simulink model "myTV_MPCC_fix"  (R2023b)
settings: Solver=VariableStepAuto  StartTime=0.0  StopTime=10.0  FixedStep=1e-6  RelTol=1e-3
libraries: spsDCVoltageSourceLib x1, slpidlib x1, spsPermanentMagnetSynchronousMachineLib x1, spsUniversalBridgeLib x1, spspowerguiLib x1
settings Model: Creator=XieXW  LastModifiedBy=XieXW
settings ModelReferenceCC: EnableRefExpFcnMdlSchedulingChecks=on

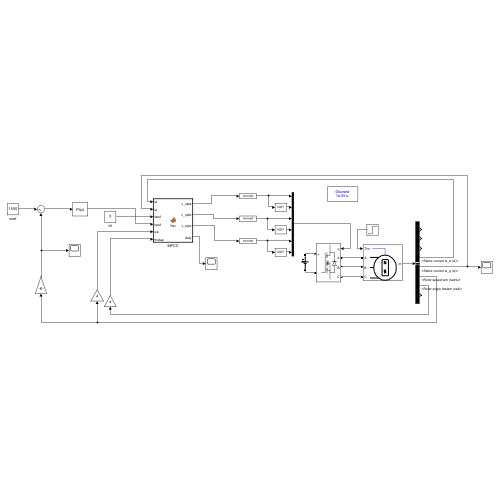
[thumbnail: Simulink's stored preview of the top-level diagram]
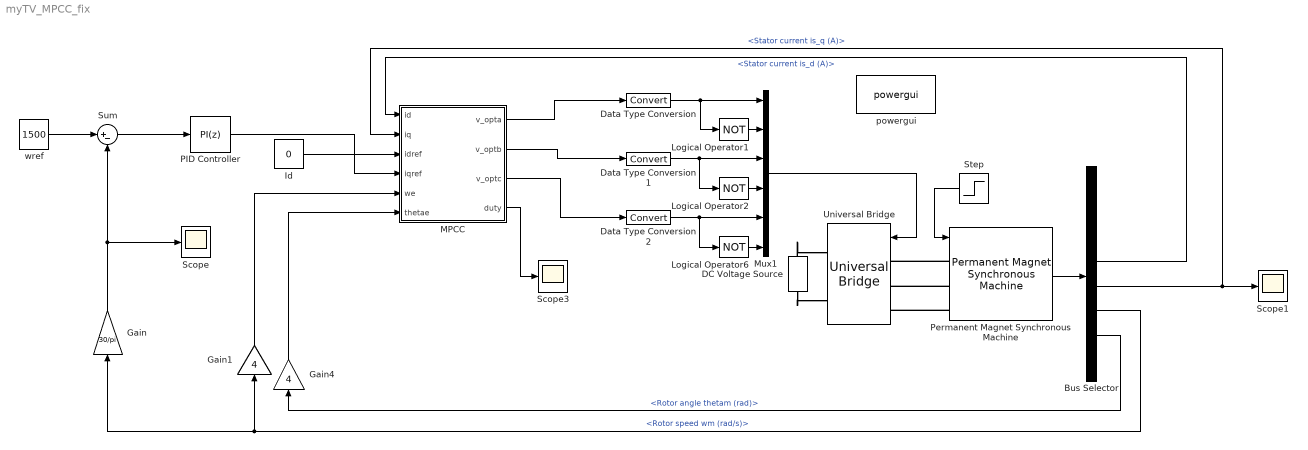
== system myTV_MPCC_fix ==
  Bus Selector : BusSelector  OutputSignals=Stator current is_a (A),Stator current is_b (A),Stator current is_c (A),Stator current is_d (A),Stator current is_q (A),Rotor speed wm (rad/s),Rotor angle thetam (rad),Electromagnetic torque Te (N*m)
  DC Voltage Source : spsDCVoltageSourceLib/DC Voltage Source  Amplitude=24  Measurements=None
  Data Type Conversion : DataTypeConversion  SaturateOnIntegerOverflow=off  RndMeth=Floor
  Data Type Conversion1 : DataTypeConversion  SaturateOnIntegerOverflow=off  RndMeth=Floor
  Data Type Conversion2 : DataTypeConversion  SaturateOnIntegerOverflow=off  RndMeth=Floor
  Gain : Gain  Gain=30/pi
  Gain1 : Gain  Gain=4
  Gain4 : Gain  Gain=4
  Id : Constant  Value=0
  Logical Operator1 : Logic  Operator=NOT  AllPortsSameDT=off  OutDataTypeStr=boolean
  Logical Operator2 : Logic  Operator=NOT  AllPortsSameDT=off  OutDataTypeStr=boolean
  Logical Operator6 : Logic  Operator=NOT  AllPortsSameDT=off  OutDataTypeStr=boolean
  MPCC : MATLAB Function  TreatAsAtomicUnit=on
  Mux1 : Mux  Inputs=6
  PID Controller : slpidlib/PID Controller  Controller=PI  Form=Parallel  TimeDomain=Discrete-time  UseExternalTs=off  SampleTime=-1  IntegratorMethod=Forward Euler  FilterMethod=Forward Euler  ControllerParametersSource=internal  P=0.6  I=0.7  UseKiTs=off  D=0  N=100  UseFilter=on  TunerSelectOption=Transfer Function Based (PID Tuner App)  InitialConditionSource=internal  InitialConditionForIntegrator=0  InitialConditionForFilter=0  DifferentiatorICPrevScaledInput=0  ExternalReset=none  TrackingMode=off  Kt=1  LimitOutput=off  SatLimitsSource=internal  UpperSaturationLimit=inf  LowerSaturationLimit=-inf  LinearizeAsGain=on  AntiWindupMode=none  Kb=1  LimitIntegrator=off  UpperIntegratorSaturationLimit=inf  LowerIntegratorSaturationLimit=-inf  POutMin=[]  POutMax=[]  IOutMin=[]  IOutMax=[]  DOutMin=[]  DOutMax=[]  NOutMin=[]  NOutMax=[]  SumOutMin=[]  SumOutMax=[]  SaturationOutMin=[]  SaturationOutMax=[]  PParamMin=[]  PParamMax=[]  IParamMin=[]  IParamMax=[]  DParamMin=[]  DParamMax=[]  NParamMin=[]  NParamMax=[]  KbParamMin=[]  KbParamMax=[]  KtParamMin=[]  KtParamMax=[]  KbOutMin=[]  KbOutMax=[]  KtOutMin=[]  KtOutMax=[]  IntegratorOutMin=[]  IntegratorOutMax=[]  FilterOutMin=[]  FilterOutMax=[]  SumI1OutMin=[]  SumI1OutMax=[]  SumI2OutMin=[]  SumI2OutMax=[]  SumI3OutMin=[]  SumI3OutMax=[]  SumI4OutMin=[]  SumI4OutMax=[]  SumDOutMin=[]  SumDOutMax=[]  DifferentiatorOutMin=[]  DifferentiatorOutMax=[]  FilterDiffOutCoefMin=[]  FilterDiffOutCoefMax=[]  ReciprocalOutMin=[]  ReciprocalOutMax=[]  SumDenOutMin=[]  SumDenOutMax=[]  SumNumOutMin=[]  SumNumOutMax=[]  DivideOutMin=[]  DivideOutMax=[]  UdiffTsProdOutMin=[]  UdiffTsProdOutMax=[]  NTsProdOutMin=[]  NTsProdOutMax=[]  UintegralTsProdOutMin=[]  UintegralTsProdOutMax=[]  UngainTsProdOutMin=[]  UngainTsProdOutMax=[]  ClampingZeroOutDataTypeStr=Inherit: Inherit via back propagation  ClampingZeroOutMin=[]  ClampingZeroOutMax=[]  FilterDenConstantOutDataTypeStr=Inherit: Inherit via back propagation  FilterDenConstantOutMin=[]  FilterDenConstantOutMax=[]  PCopyOutDataTypeStr=Inherit: Inherit via back propagation  PCopyOutMin=[]  PCopyOutMax=[]  NCopyOutDataTypeStr=Inherit: Inherit via back propagation  NCopyOutMin=[]  NCopyOutMax=[]  IntegratorContinuousStateAttributes=''  IntegratorStateMustResolveToSignalObject=off  IntegratorRTWStateStorageClass=Auto  FilterContinuousStateAttributes=''  FilterStateMustResolveToSignalObject=off  FilterRTWStateStorageClass=Auto  ParallelPVariant=InternalParameters  IdealPVariant=Disabled  IVariant=InternalParameters  DVariant=Disabled  IntegratorVariant=Discrete  SatVariant=Disabled  AWVariant=Passthrough  PCopyVariant=Disabled  TRVariant=Disabled  FdbkBlocksVariant=Forward  IdealPFdbkVariant=Disabled  SatFdbkVariant=Disabled  DerivativeFilterVariant=Disabled  NVariant=Disabled  NCopyVariant=Disabled_SignalSpec  FilterICVariant=Disabled  IntegratorICVariant=InternalICs  ExternalResetVariant=Disabled  TRSumVariant=Passthrough  SumFdbkVariant=Disabled  SumVariant=Sum_PI  TsampFilterVariant=InternalTs  TsampNgainVariant=Passthrough  TsampIntegralVariant=Disabled_SignalSpec  ExternalSaturationOutDataTypeStr=Inherit: Same as second input
  Permanent Magnet Synchronous Machine : spsPermanentMagnetSynchronousMachineLib/Permanent Magnet Synchronous Machine  NbPhases=3  FluxDistribution=Sinusoidal  RotorType=Round  MechanicalLoad=Torque Tm  PresetModel=No  ShowDetailedParameters=on  MeasurementBus=off  Resistance=0.03  Inductance=8.5e-3  dqInductances=[8.5e-3,8.5e-3]  La=0.00015  MachineConstant=Flux linkage established by magnets (V.s)  Flux=0.008  VoltageCst=5.8042  TorqueCst=0.048  Flat=120  Mechanical=[0.0027 0.0004924 4 0]  PolePairs=4  InitialConditions=[0,0, 0,0]  InitialConditions5ph=[0 0 0 0 0 0]  RefAngle=Aligned with phase A axis (original Park)  IterativeDiscreteModel=Trapezoidal non iterative  TsBlock=-1  TsPowergui=0
  Scope : Scope
  Scope1 : Scope
  Scope3 : Scope
  Step : Step  Time=5  After=2  SampleTime=0
  Sum : Sum  Inputs=|+-
  Universal Bridge : spsUniversalBridgeLib/Universal Bridge  Arms=3  SnubberResistance=1e5  SnubberCapacitance=inf  Device=MOSFET / Diodes  Ron=1e-3  Lon=0  ForwardVoltages="[  0  0  ]"  ForwardVoltage=0  GTOparameters=[ 10e-6 , 20e-6 ]  IGBTparameters=[ 1e-6 , 2e-6 ]  Measurements=None  Measurements_2=None  converterType=Rectifier
  powergui : spspowerguiLib/powergui  Priority=1  SimulationMode=Discrete  SampleTime=1e-05  frequency=60  Iterations=50  frequencyindice=0  Pbase=100e6  ErrMax=1e-4  UnitsV=kV  UnitsW=MW  buscounter=0  FunctionMessages=off  echomessages=off  EnableUseOfTLC=off  CurrentSourceSwitches=off  DisableSnubberDevices=off  DisableRonSwitches=off  DisableVfSwitches=off  DisplayEquations=off  AutomaticDiscreteSolvers=off  SolverType=Tustin/Backward Euler (TBE)  Interpol=off  ExternalGateDelay=off  methode=off  Ts=100  x0status=blocks  SPID=on  SwTol=0  HookPort=off  NonlinearTolerance=1e-4  nMaxIteration=100  ContinueOnMaxIteration=off  RestoreLinks=warning  ResistiveCurrentMeasurement=off  Frange=[0:2:500]  Ylog=off  Xlog=on  ShowGrid=off  save=off  variable=ZData  structure=0  ZoomFFT=off  StartTime=0.0  cycles=1  DisplayStyle=1  fundamental=60  FreqAxis=off  MaxFrequency=1000  frequencyindicesteady=1  RmsSteady=1  display=off
  wref : Constant  Value=1500
  wires:
  wref/1 -> Sum/1
  Sum/1 -> PID Controller/1
  PID Controller/1 -> MPCC/4(iqref)
  Permanent Magnet Synchronous Machine/1 -> Bus Selector/1
  Bus Selector/4 -> MPCC/1(id)  "<Stator current is_d (A)>"
  Bus Selector/5 -> Scope1/1, MPCC/2(iq)  "<Stator current is_q (A)>"
  Bus Selector/7 -> Gain4/1  "<Rotor angle thetam (rad)>"
  Bus Selector/6 -> Gain/1, Gain1/1  "<Rotor speed wm (rad/s)>"
  Id/1 -> MPCC/3(idref)
  Gain/1 -> Sum/2, Scope/1
  Gain4/1 -> MPCC/6(thetae)
  Gain1/1 -> MPCC/5(we)
  Step/1 -> Permanent Magnet Synchronous Machine/1
  MPCC/2(v_optb) -> Data Type Conversion1/1
  Logical Operator6/1 -> Mux1/6
  Data Type Conversion/1 -> Mux1/1, Logical Operator1/1
  Logical Operator1/1 -> Mux1/2
  Mux1/1 -> Universal Bridge/1
  MPCC/1(v_opta) -> Data Type Conversion/1
  Logical Operator2/1 -> Mux1/4
  Data Type Conversion1/1 -> Mux1/3, Logical Operator2/1
  MPCC/4(duty) -> Scope3/1
  Data Type Conversion2/1 -> Logical Operator6/1, Mux1/5
  MPCC/3(v_optc) -> Data Type Conversion2/1
  connections:
  Permanent Magnet Synchronous Machine/LConn1 -- Universal Bridge/LConn1
  Permanent Magnet Synchronous Machine/LConn2 -- Universal Bridge/LConn2
  Permanent Magnet Synchronous Machine/LConn3 -- Universal Bridge/LConn3
  DC Voltage Source/RConn1 -- Universal Bridge/RConn1
  DC Voltage Source/LConn1 -- Universal Bridge/RConn2

== matlab function myTV_MPCC_fix/MPCC ==
  settings: sampleTime=20e-6
  data: id input; v_opta output; v_optb output; v_optc output; duty output; iq input; idref input; iqref input; we input; thetae input
function [v_opta,v_optb,v_optc,duty] = fcn(id,iq,idref,iqref,we,thetae)

Rs=0.03;
Ls=0.00015;
psif=0.008;
vdc=24;
Ts=1e-4;
set=[0 0 0;0 1 0;0 0 1;0 1 1;1 0 0;1 0 1;1 1 0];%电压矢量开关集合
cost = 1000000;
state1 = 1;
state2 = 1;
%%开始计算第一个最优电压矢量
for i=1:7
    udi=2/3*vdc*( set(i,1)*cos(thetae)+set(i,2)*cos(thetae-2*pi/3)+set(i,3)*cos(thetae+2*pi/3));
    uqi=2/3*vdc*(-set(i,1)*sin(thetae)-set(i,2)*sin(thetae-2*pi/3)-set(i,3)*sin(thetae+2*pi/3));
    id1 = id+Ts/Ls*(udi-Rs*id+we*Ls*iq);
    iq1 = iq+Ts/Ls*(uqi-Rs*iq-we*(Ls*id+psif));

    J = (idref-id1)^2+(iqref-iq1)^2;
    if J<cost
        state1=i;
        cost = J;
    end

end
%%第一个最优电压矢量
v_opt1_a = set(state1,1);
v_opt1_b = set(state1,2);
v_opt1_c = set(state1,3);
v_opt1 = [v_opt1_a,v_opt1_b,v_opt1_c];

%%开始计算第二个最优电压矢量
%计算最优电压矢量
uq_opt1 = 2/3*vdc*( set(state1,1)*cos(thetae)+set(state1,2)*cos(thetae-2*pi/3)+set(state1,3)*cos(thetae+2*pi/3));
ud_opt1 = 2/3*vdc*(-set(state1,1)*sin(thetae)-set(state1,2)*sin(thetae-2*pi/3)-set(state1,3)*sin(thetae+2*pi/3));

slope = [0 0 0 0 0 0 0];                %七个电压矢量作用下的q轴电流斜率
slope_0 = -Rs/Ls*iq-we*id-we*psif/Ls;    %零电压矢量作用下的q轴电流斜率
slope_opt = slope_0 + uq_opt1/Ls;       %最优矢量作用下的q轴电流斜率

%重新初始化代价值
cost = 1000000;

for j=1:7
    %%步骤1
    %计算第j个电压矢量的dq轴分量,对应论文中的uqj、udj
    udj=2/3*vdc*( set(j,1)*cos(thetae)+set(j,2)*cos(thetae-2*pi/3)+set(j,3)*cos(thetae+2*pi/3));
    uqj=2/3*vdc*(-set(j,1)*sin(thetae)-set(j,2)*sin(thetae-2*pi/3)-set(j,3)*sin(thetae+2*pi/3));
    
    slope(j)=slope_0 + uqj/Ls;
    t_opt1 = (iqref-iq-slope(j)*Ts)/(slope_opt-slope(j));
    t_opt2 = Ts - t_opt1;
    %%步骤2
    %计算dq轴电压,对应原文公式(12),(13)
    uq = t_opt1*uq_opt1 + t_opt2*uqj;
    ud = t_opt1*ud_opt1 + t_opt2*udj;
    
    id2 = id+Ts/Ls*(ud-Rs*id+we*Ls*iq);
    iq2 = iq+Ts/Ls*(uq-Rs*iq-we*(Ls*id+psif));

    %%步骤3
    J = (idref-id2)^2+(iqref-iq2)^2;
    if J<cost
        state2 = j;
        cost = J;
    end
end
%%第二个最优电压矢量
v_opt2_a = set(state2,1);
v_opt2_b = set(state2,2);
v_opt2_c = set(state2,3);
% v_opt2 = [v_opt2_a,v_opt2_b,v_opt2_c];

duty = t_opt1/Ts;

v_opta = v_opt1_a*t_opt1 + v_opt2_a *t_opt2;
v_optb = v_opt1_b*t_opt1 + v_opt2_b *t_opt2;
v_optc = v_opt1_c*t_opt1 + v_opt2_c *t_opt2;

end
